simulink model "CTRL_LO_ST1_TRQDMDWHL_test"  (R2023b)
settings: Solver=VariableStepAuto  StartTime=0.0  StopTime=10.0  RelTol=1e-3
libraries: CTRL_LO_ST1_TRQDMDWHL x1
settings Model: Creator=blatak  LastModifiedBy=blatak

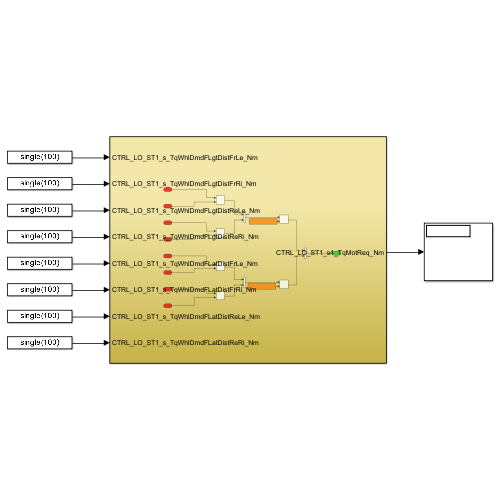
[thumbnail: Simulink's stored preview of the top-level diagram]
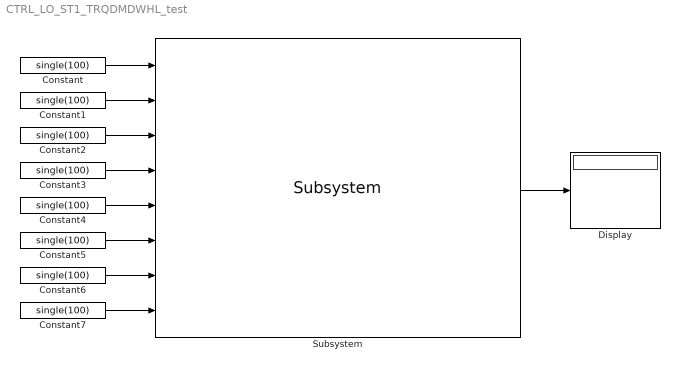
== system CTRL_LO_ST1_TRQDMDWHL_test ==
  Constant{,1..7} (8 alike) : Constant  Value=single(100)
  Display : Display
  Subsystem : CTRL_LO_ST1_TRQDMDWHL/Subsystem  SystemSampleTime=-1  VariantActivationTime=update diagram  AllowFlexibleInterface=on  Latency=0  AutoFrameSizeCalculation=off
  wires:
  Constant/1 -> Subsystem/1
  Constant1/1 -> Subsystem/2
  Constant2/1 -> Subsystem/3
  Constant3/1 -> Subsystem/4
  Constant4/1 -> Subsystem/5
  Constant5/1 -> Subsystem/6
  Constant6/1 -> Subsystem/7
  Constant7/1 -> Subsystem/8
  Subsystem/1 -> Display/1
